simulink model "floatingBase_fourLinks_DynamicModel"  (R2022a)
settings: Solver=FixedStepAuto  StartTime=0  StopTime=100  FixedStep=0.1  RelTol=1e-3
InitFcn:
  | Init_data
values from neighbouring files (symbols this model uses):
  dq0 = 0    [Init_data.m]
  dqm = [0,0,0,0].'    [Init_data.m]
  Kdbf = 5    [Init_data.m]
  Kdmf = diag([10,15,10,15])    [Init_data.m]
  Kibc = 1    [Init_data.m]
  Kimc = diag([1,1,1,1])    [Init_data.m]
  Kpbc = 1    [Init_data.m]
  Kpbf = 10    [Init_data.m]
  Kpmc = diag([1,1,1,1])    [Init_data.m]
  Kpmf = diag([1,1,1,1])    [Init_data.m]
  q0 = 0.3    [Init_data.m]    (also in calc_Mass.m = w0)
  q0_d = 0    [Init_data.m]
  qm = [0.1,0.15,0.25,0.3].'    [Init_data.m]
  qm_d = [0,0,0,0].'    [Init_data.m]
settings Model: Creator=43840  LastModifiedBy=43840

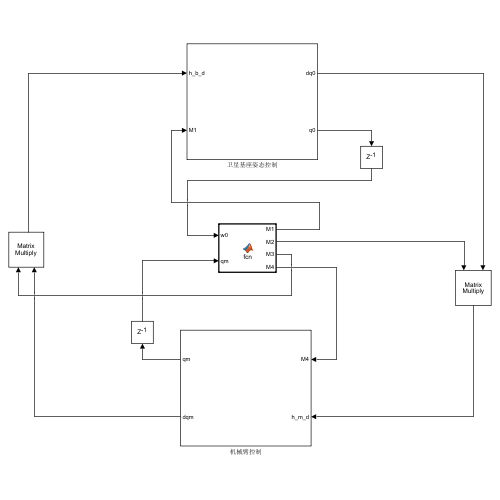
[thumbnail: Simulink's stored preview of the top-level diagram]
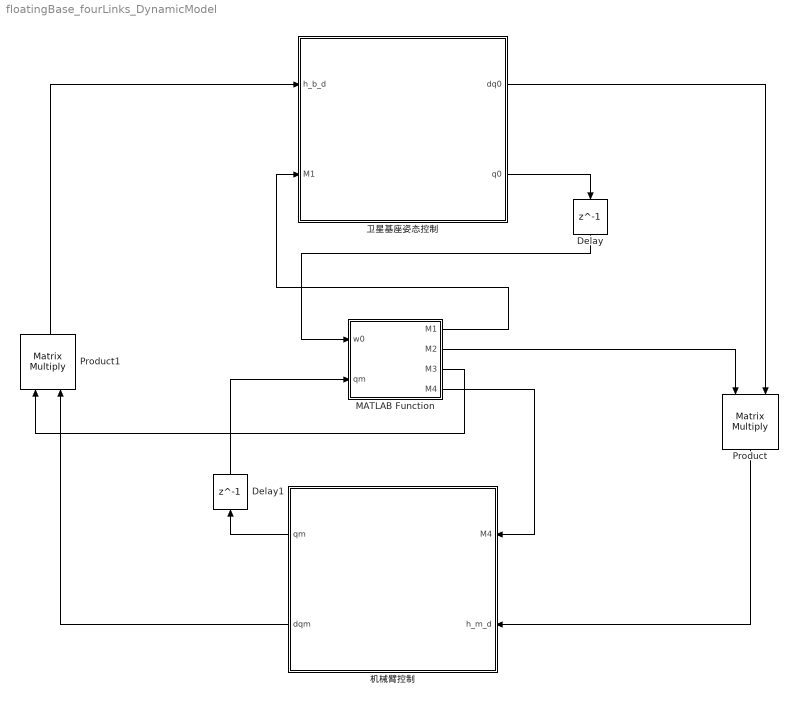
== system floatingBase_fourLinks_DynamicModel ==
  Delay : Delay  DelayLength=1
  Delay1 : Delay  DelayLength=1
  MATLAB Function : MATLAB Function  TreatAsAtomicUnit=on
  Product : Product  Multiplication=Matrix(*)
  Product1 : Product  Multiplication=Matrix(*)
  卫星基座姿态控制 : Subsystem
  机械臂控制 : Subsystem
  wires:
  Product1/1 -> 卫星基座姿态控制/1(h_b_d)
  机械臂控制/2(dqm) -> Product1/2
  Product/1 -> 机械臂控制/2(h_m_d)
  卫星基座姿态控制/1(dq0) -> Product/2
  机械臂控制/1(qm) -> Delay1/1
  卫星基座姿态控制/2(q0) -> Delay/1
  MATLAB Function/1(M1) -> 卫星基座姿态控制/2(M1)
  MATLAB Function/4(M4) -> 机械臂控制/1(M4)
  MATLAB Function/2(M2) -> Product/1
  MATLAB Function/3(M3) -> Product1/1
  Delay/1 -> MATLAB Function/1(w0)
  Delay1/1 -> MATLAB Function/2(qm)

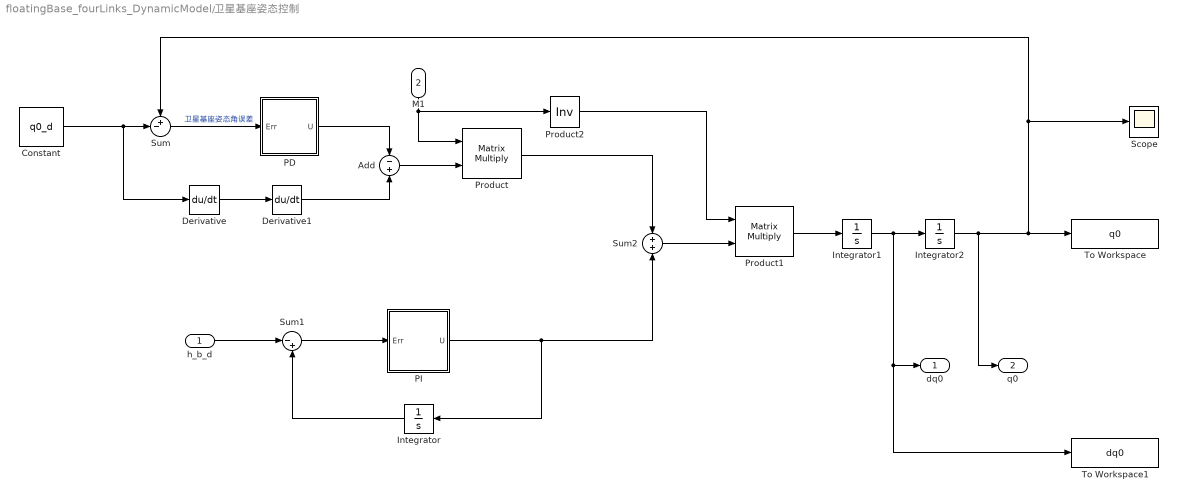
== system floatingBase_fourLinks_DynamicModel/卫星基座姿态控制 ==
  h_b_d : Inport
  M1 : Inport  Port=2
  Add : Sum  Inputs=-+
  Constant : Constant  Value=q0_d  VectorParams1D=off
  Derivative : Derivative
  Derivative1 : Derivative
  Integrator : Integrator
  Integrator1 : Integrator  InitialCondition=dq0
  Integrator2 : Integrator  InitialCondition=q0
  PD : Subsystem
  PI : Subsystem
  Product : Product  Multiplication=Matrix(*)
  Product1 : Product  Multiplication=Matrix(*)
  Product2 : Product  Inputs=/  Multiplication=Matrix(*)
  Scope : Scope
  Sum : Sum  Inputs=+-|
  Sum1 : Sum  Inputs=|-+
  Sum2 : Sum  Inputs=+|+
  To Workspace : ToWorkspace  VariableName=q0  SampleTime=-1
      settings: Save2DSignal=2-D array (concatenate along first dimension)
  To Workspace1 : ToWorkspace  VariableName=dq0  SampleTime=-1
      settings: Save2DSignal=2-D array (concatenate along first dimension)
  dq0 : Outport
  q0 : Outport  Port=2
  wires:
  Sum/1 -> PD/1(Err)  "卫星基座姿态角误差"
  Integrator/1 -> Sum1/2
  Sum1/1 -> PI/1(Err)
  Derivative/1 -> Derivative1/1
  Product/1 -> Sum2/1
  PD/1(U) -> Add/1
  Add/1 -> Product/2
  PI/1(U) -> Sum2/2, Integrator/1
  h_b_d/1 -> Sum1/1
  Integrator1/1 -> Integrator2/1, To Workspace1/1, dq0/1
  Derivative1/1 -> Add/2
  Constant/1 -> Derivative/1, Sum/2
  Integrator2/1 -> q0/1, To Workspace/1, Scope/1, Sum/1
  M1/1 -> Product2/1, Product/1
  Product2/1 -> Product1/1
  Product1/1 -> Integrator1/1
  Sum2/1 -> Product1/2

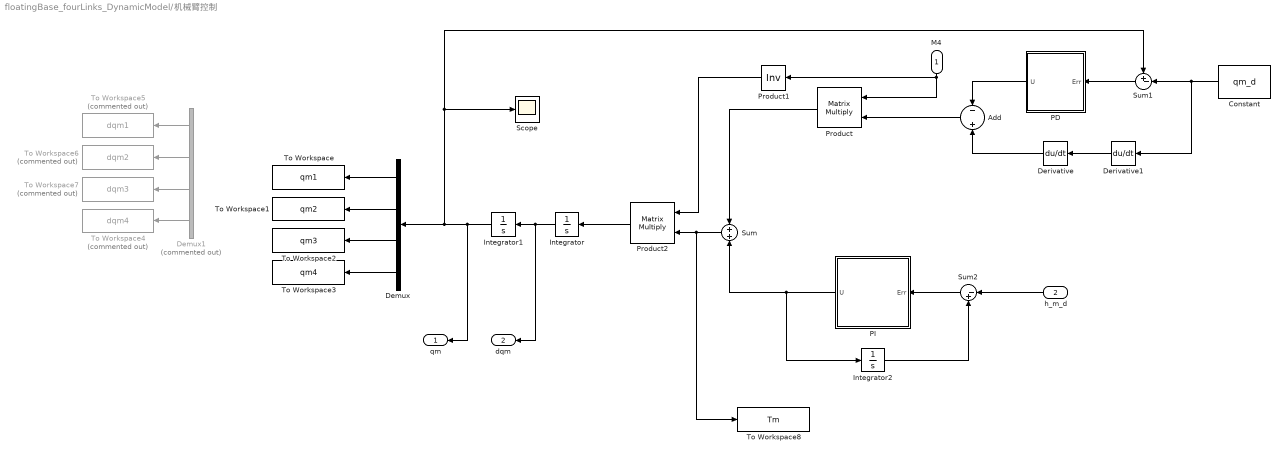
== system floatingBase_fourLinks_DynamicModel/机械臂控制 ==
  M4 : Inport
  h_m_d : Inport  Port=2
  Add : Sum  Inputs=-+
  Constant : Constant  Value=qm_d
  Demux : Demux
  Demux1 : Demux  Commented=on
  Derivative : Derivative
  Derivative1 : Derivative
  Integrator : Integrator  InitialCondition=dqm
  Integrator1 : Integrator  InitialCondition=qm
  Integrator2 : Integrator
  PD : Subsystem
  PI : Subsystem
  Product : Product  Multiplication=Matrix(*)
  Product1 : Product  Inputs=/  Multiplication=Matrix(*)
  Product2 : Product  Multiplication=Matrix(*)
  Scope : Scope
  Sum : Sum
  Sum1 : Sum  Inputs=+-|
  Sum2 : Sum  Inputs=|-+
  To Workspace : ToWorkspace  VariableName=qm1  SampleTime=-1
      settings: Save2DSignal=2-D array (concatenate along first dimension)
  To Workspace1 : ToWorkspace  VariableName=qm2  SampleTime=-1
      settings: Save2DSignal=2-D array (concatenate along first dimension)
  To Workspace2 : ToWorkspace  VariableName=qm3  SampleTime=-1
      settings: Save2DSignal=2-D array (concatenate along first dimension)
  To Workspace3 : ToWorkspace  VariableName=qm4  SampleTime=-1
      settings: Save2DSignal=2-D array (concatenate along first dimension)
  To Workspace4 : ToWorkspace  Commented=on  VariableName=dqm4  SampleTime=-1
      settings: Save2DSignal=2-D array (concatenate along first dimension)
  To Workspace5 : ToWorkspace  Commented=on  VariableName=dqm1  SampleTime=-1
      settings: Save2DSignal=2-D array (concatenate along first dimension)
  To Workspace6 : ToWorkspace  Commented=on  VariableName=dqm2  SampleTime=-1
      settings: Save2DSignal=2-D array (concatenate along first dimension)
  To Workspace7 : ToWorkspace  Commented=on  VariableName=dqm3  SampleTime=-1
      settings: Save2DSignal=2-D array (concatenate along first dimension)
  To Workspace8 : ToWorkspace  VariableName=Tm  SampleTime=-1
  qm : Outport
  dqm : Outport  Port=2
  wires:
  Integrator2/1 -> Sum2/2
  PI/1(U) -> Sum/2, Integrator2/1
  Sum2/1 -> PI/1(Err)
  Product2/1 -> Integrator/1
  Constant/1 -> Sum1/2, Derivative1/1
  Derivative1/1 -> Derivative/1
  Sum1/1 -> PD/1(Err)
  Product/1 -> Sum/1
  Add/1 -> Product/2
  PD/1(U) -> Add/1
  Derivative/1 -> Add/2
  h_m_d/1 -> Sum2/1
  Demux/1 -> To Workspace/1
  Demux/2 -> To Workspace1/1
  Demux/3 -> To Workspace2/1
  Demux/4 -> To Workspace3/1
  M4/1 -> Product/1, Product1/1
  Integrator/1 -> dqm/1, Integrator1/1
  Demux1/1 -> To Workspace5/1
  Demux1/2 -> To Workspace6/1
  Demux1/3 -> To Workspace7/1
  Demux1/4 -> To Workspace4/1
  Product1/1 -> Product2/1
  Sum/1 -> To Workspace8/1, Product2/2
  Integrator1/1 -> qm/1, Demux/1, Scope/1, Sum1/1

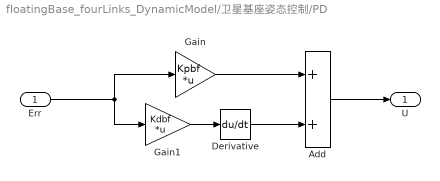
== system floatingBase_fourLinks_DynamicModel/卫星基座姿态控制/PD ==
  Err : Inport
  Add : Sum
  Derivative : Derivative
  Gain : Gain  Gain=Kpbf  Multiplication=Matrix(K*u)
  Gain1 : Gain  Gain=Kdbf  Multiplication=Matrix(K*u)
  U : Outport
  wires:
  Err/1 -> Gain1/1, Gain/1
  Gain1/1 -> Derivative/1
  Gain/1 -> Add/1
  Derivative/1 -> Add/2
  Add/1 -> U/1

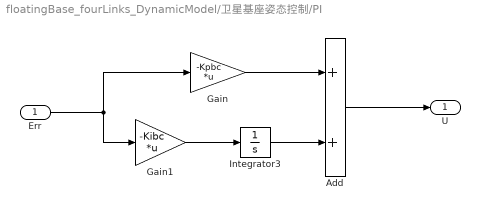
== system floatingBase_fourLinks_DynamicModel/卫星基座姿态控制/PI ==
  Err : Inport
  Add : Sum
  Gain : Gain  Gain=-Kpbc  Multiplication=Matrix(K*u)
  Gain1 : Gain  Gain=-Kibc  Multiplication=Matrix(K*u)
  Integrator3 : Integrator
  U : Outport
  wires:
  Gain1/1 -> Integrator3/1
  Add/1 -> U/1
  Gain/1 -> Add/1
  Err/1 -> Gain1/1, Gain/1
  Integrator3/1 -> Add/2

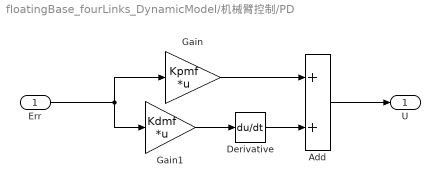
== system floatingBase_fourLinks_DynamicModel/机械臂控制/PD ==
  Err : Inport
  Add : Sum
  Derivative : Derivative
  Gain : Gain  Gain=Kpmf  Multiplication=Matrix(K*u)
  Gain1 : Gain  Gain=Kdmf  Multiplication=Matrix(K*u)
  U : Outport
  wires:
  Err/1 -> Gain1/1, Gain/1
  Gain1/1 -> Derivative/1
  Gain/1 -> Add/1
  Derivative/1 -> Add/2
  Add/1 -> U/1

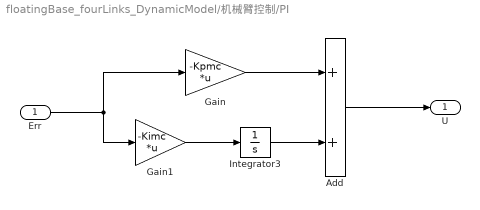
== system floatingBase_fourLinks_DynamicModel/机械臂控制/PI ==
  Err : Inport
  Add : Sum
  Gain : Gain  Gain=-Kpmc  Multiplication=Matrix(K*u)
  Gain1 : Gain  Gain=-Kimc  Multiplication=Matrix(K*u)
  Integrator3 : Integrator
  U : Outport
  wires:
  Gain1/1 -> Integrator3/1
  Add/1 -> U/1
  Gain/1 -> Add/1
  Err/1 -> Gain1/1, Gain/1
  Integrator3/1 -> Add/2

== matlab function floatingBase_fourLinks_DynamicModel/MATLAB Function ==
  data: w0 input; M1 output; qm input; M2 output; M3 output; M4 output
function [M1, M2, M3, M4] = fcn(w0,qm)

coder.extrinsic("calc_Mass")

M1=zeros(1,1);
M2=zeros(4,1);
M3=zeros(1,4);
M4=zeros(4,4);

[M1, M2, M3, M4]=calc_Mass(w0,qm);
